simulink model "Lab4_1"  (R2024a)
settings: Solver=VariableStepAuto  StartTime=0.0  StopTime=100  RelTol=1e-3
libraries: dspsrcs4 x1
settings Model: Creator=user  LastModifiedBy=user

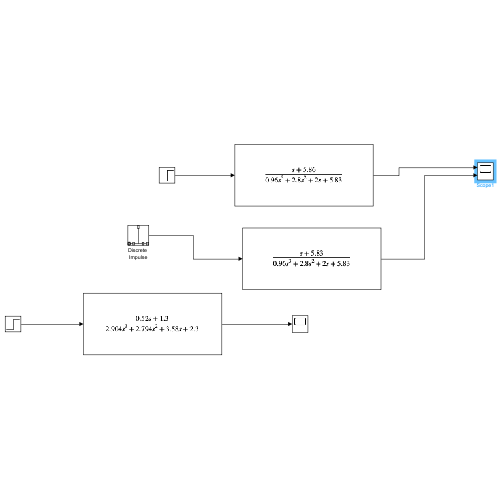
[thumbnail: Simulink's stored preview of the top-level diagram]
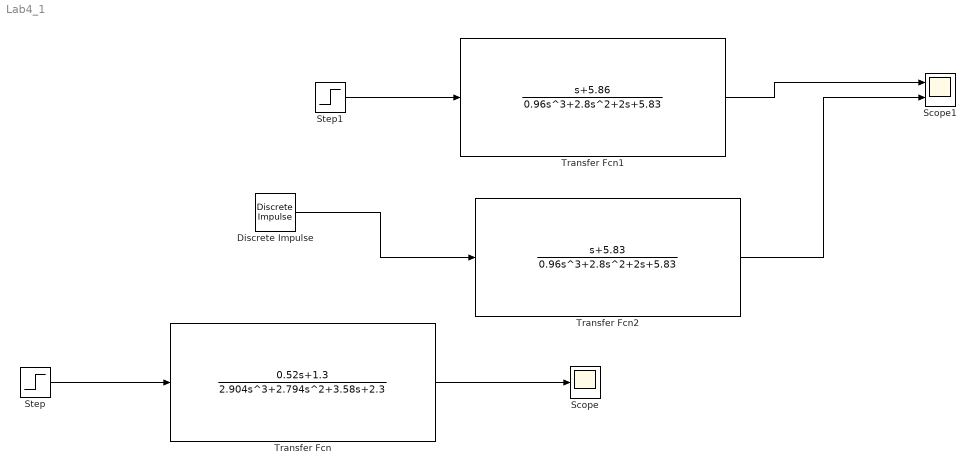
== system Lab4_1 ==
  Discrete Impulse : dspsrcs4/Discrete  Impulse  Delay=0  SampleTime=1  FrameSample=1  OutputFrames=off  dataType=double  isSigned=on  wordLen=16  udDataType=sfix(16)  fracBitsMode=Best precision  numFracBits=15  OutDataTypeStr=double  LastOutDataTypeStr=double
  Scope : Scope
  Scope1 : Scope  NumInputPorts=2
  Step : Step  SampleTime=0
  Step1 : Step  SampleTime=0
  Transfer Fcn : TransferFcn  Numerator=[0.52 1.3]  Denominator=[2.904 2.794 3.58 2.3]
  Transfer Fcn1 : TransferFcn  Numerator=[1 5.86]  Denominator=[0.96 2.8 2 5.83]  ParameterTunability=Optimized
  Transfer Fcn2 : TransferFcn  Numerator=[1 5.83]  Denominator=[0.96 2.8 2 5.83]  ParameterTunability=Optimized
  wires:
  Transfer Fcn/1 -> Scope/1
  Step/1 -> Transfer Fcn/1
  Step1/1 -> Transfer Fcn1/1
  Transfer Fcn1/1 -> Scope1/1
  Discrete Impulse/1 -> Transfer Fcn2/1
  Transfer Fcn2/1 -> Scope1/2
